simulink model "HalfBandInterpolator_Ex2"  (R2025a)
settings: Solver=VariableStepAuto  StopTime=1
InitFcn:
  | HalfBandInterpolator = 4*firhalfband('minorder', 10e3/(100e3/2), 5.7564627261e-05);
  | FilterCoefficients = HalfBandInterpolator([1:2:(length(HalfBandInterpolator)-1)/2 (length(HalfBandInterpolator)+1)/2]);
undefined symbols (not defined in the file): firhalfband, None, S, vsva2197, xcvc1902
libraries: dspsrcs4 x1, aieDSP x1, dspmlti4 x1, vmcUtilities x1
settings Model: Creator=sdegala  LastModifiedBy=robg
settings ModelReferenceCC: EnableRefExpFcnMdlSchedulingChecks=on
settings RTWCC: GPUComputeCapability=3.5

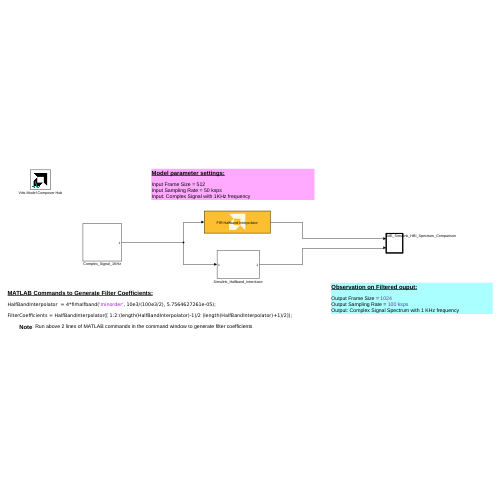
[thumbnail: Simulink's stored preview of the top-level diagram]
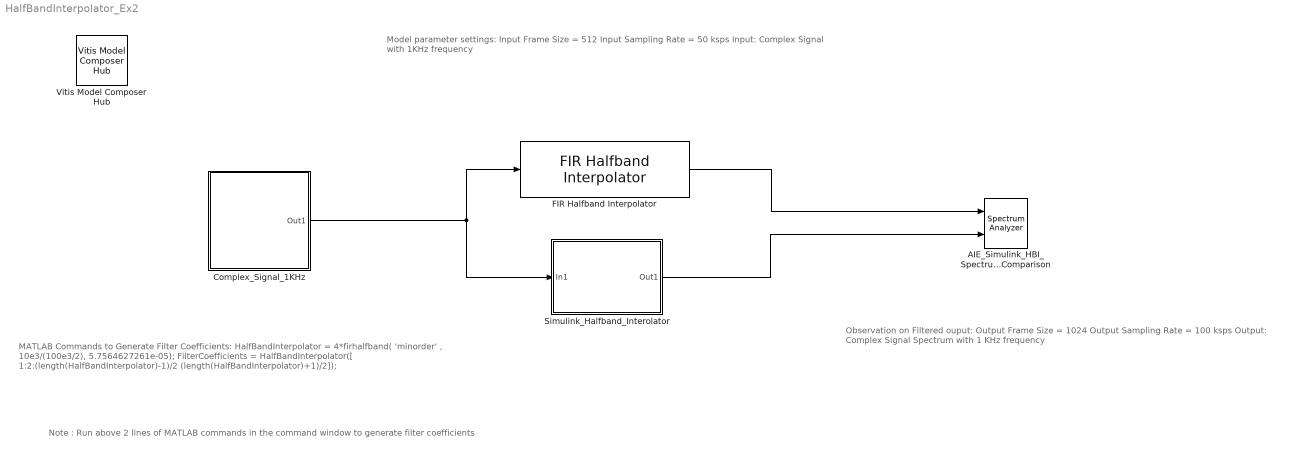
== system HalfBandInterpolator_Ex2 ==
  note: Model parameter settings:
      |
      | Input Frame Size = 512
      | Input Sampling Rate = 50 ksps
      | Input: Complex Signal with 1KHz frequency
  note: MATLAB Commands to Generate Filter Coefficients:
      |
      | HalfBandInterpolator = 4*firhalfband( 'minorder' , 10e3/(100e3/2), 5.7564627261e-05);
      |
      | FilterCoefficients = HalfBandInterpolator([ 1:2:(length(HalfBandInterpolator)-1)/2 (length(HalfBandInterpolator)+1)/2]);
  note: Note : Run above 2 lines of MATLAB commands in the command window to generate filter coefficients
  note: Observation on Filtered ouput:
      |
      | Output Frame Size = 1024
      | Output Sampling Rate = 100 ksps
      | Output: Complex Signal Spectrum with 1 KHz frequency
  AIE_Simulink_HBI_Spectrum_Comparison : SpectrumAnalyzer  NumInputPorts=2  AveragingMethod=Exponential  ShowLegend=on  ChannelNames="[\"\"]"  AllowFFTLengthLessThanSamplesPerUpdate=on  DefaultConfigurationName=spbscopes.SpectrumAnalyzerBlockCfg
  Complex_Signal_1KHz : Subsystem
  FIR Halfband Interpolator : aieDSP/FIR Halfband Interpolator  data_type=cfloat  coef_type=float  use_coeff_reload=off  dual_ip=off  num_outputs=off  coeff=FilterCoefficients  fir_length=31  input_window_size=512  shift_val=0  rnd_mode=Round to positive infinity  sat_mode=0-None  interp_poly=1  upshift_ct=off  casc_length=1  AIE_VARIANT=1  TP_API=0  ssr=1  blockJsonConstraints=[]  blockJsonConstraintsInternal=[]  spec=vmc_fir_interpolate_hb.json  SerializedMaskParamNames=[]  SerializedMaskParamValues=[]  SerializedMaskParamVisibilities=[]  block_type=FIR Halfband Interpolator  SerializedMaskParamDataypes=typename|typename|uint|uint|uint|coef_type|uint|uint|uint|uint|uint|uint|uint|uint|uint|uint|uint  SerializedMaskParamEnumStrArr=0|0|0|0|0|0|0|0|0|Floor,Ceiling,Round to positive infinity,Round to negative infinity,Round symmetrical to infinity,Round symmetrical to zero,Round convergent to even,Round convergent to odd|0-None,1-Asymmetric,3-Symmetric|0|0|0|0|0|0  SerializedMaskParamEnumValArr=0|0|0|0|0|0|0|0|0|0,1,2,3,4,5,6,7|0,1,3|0|0|0|0|0|0  SerializedMaskParamVectorArr=0|0|0|0|0|1|0|0|0|0|0|0|0|0|0|0|0  SerializedMaskParamKeys=TT_DATA|TT_COEFF|TP_USE_COEFF_RELOAD|TP_DUAL_IP|TP_NUM_OUTPUTS|coeff|TP_FIR_LEN|TP_INPUT_WINDOW_VSIZE|TP_SHIFT|TP_RND|TP_SAT|TP_PARA_INTERP_POLY|TP_UPSHIFT_CT|TP_CASC_LEN|AIE_VARIANT|TP_API|TP_SSR
  Simulink_Halfband_Interolator : Subsystem
  Vitis Model Composer Hub : vmcUtilities/Vitis Model Composer Hub  Tag=genX  CodeGeneration=off  StartColumn=1  NumberOfColumns=1  TargetDirectory=./code  exportDesign=off  analyzeDesign=off  validateDesignOnHw=off  ExportType=AI Engines  IpVendor=xilinx.com  IpLibrary=hls  IpVersion=1.0  IpHWLanguage=Verilog  AieCompilerOptions={}  AieSimulatorOptions={}  CreateTestbench=off  TestbenchStackSize=10  RunRtlSim=off  RunCSim=off  RunAieSim=off  enableSimulationTimeout=on  enableGraphIterations=on  AieSimTimeout=50000  AieGraphIterations=-1  RunAieSimProfiling=off  LaunchVitisAnalyzer=off  PlotOutput=off  RunX86Sim=off  X86SimTimeout=10  GenHwImage=off  GenLibadfXo=off  GenHwValidationCode=off  PlatformType=Not Specified  HwSystemType=Baremetal  HwValidationTarget=hw  ProjDevice=xcvc1902-vsva2197-1LP-e-S  ProjDevicePart=xcvc1902-vsva2197-1LP-e-S  AIEType=AIE  SamplePeriod=-1  ClockFrequency=200  DataPathParallelism=1  xilinxfamily=versalaicore  part=xcvc1902  speed=-1LP-e-S  package=vsva2197  directory=./netlist  testbench=off  incr_netlist=off  synthesis_tool=Vivado  clock_wrapper=Clock Enables  dbl_ovrd=According to Block Masks  dcm_input_clock_period=10  sysclk_period=10  simulink_period=1  eval_field=0  LogFileName=''  NThreads=4
  wires:
  FIR Halfband Interpolator/1 -> AIE_Simulink_HBI_Spectrum_Comparison/1
  Simulink_Halfband_Interolator/1(Out1) -> AIE_Simulink_HBI_Spectrum_Comparison/2
  Complex_Signal_1KHz/1(Out1) -> FIR Halfband Interpolator/1, Simulink_Halfband_Interolator/1(In1)

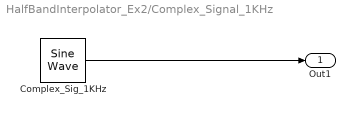
== system HalfBandInterpolator_Ex2/Complex_Signal_1KHz ==
  Complex_Sig_1KHz : dspsrcs4/Sine Wave  Amplitude=1  Frequency=1e3  Phase=0  SampleMode=Discrete  OutComplex=Complex  CompMethod=Trigonometric fcn  TableSize=Speed  SampleTime=1/50e3  SamplesPerFrame=512  ResetState=Restart at time zero  OutputFrames=off  dataType=single  wordLen=16  udDataType=sfix(16)  fracBitsMode=Best precision  numFracBits=15  OutDataTypeStr=single  LastOutDataTypeStr=single
  Out1 : Outport
  wires:
  Complex_Sig_1KHz/1 -> Out1/1

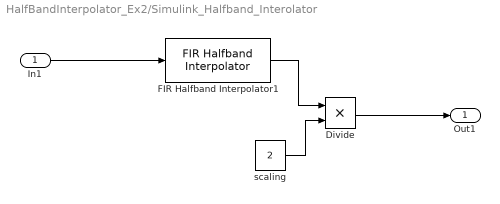
== system HalfBandInterpolator_Ex2/Simulink_Halfband_Interolator ==
  In1 : Inport
  Divide : Product  Inputs=**
  FIR Halfband Interpolator1 : dspmlti4/FIR Halfband Interpolator  Specification=Coefficients  FilterOrder=14  TransitionWidth=4.1e3  StopbandAttenuation=80  DesignMethod=Auto  Numerator=2*firhalfband('minorder', 10e3/(100e3/2), 5.7564627261e-05)  FilterBankInputPort=off  SampleRate=50e3  SimulateUsing=Code generation  roundingMode=Floor  coeffsDataTypeStr=fixdt(1,32,0)
  scaling : Constant  Value=2  OutDataTypeStr=single
  Out1 : Outport
  wires:
  FIR Halfband Interpolator1/1 -> Divide/1
  Divide/1 -> Out1/1
  scaling/1 -> Divide/2
  In1/1 -> FIR Halfband Interpolator1/1
